simulink model "untitled"  (R2020a)
settings: Solver=VariableStepAuto  StartTime=0.0  StopTime=10.0  FixedStep=1e-10  RelTol=1e-3
libraries: powerlib x18, fuzblock x1, powerlib_meascontrol x1, re_lib x1
settings Model: Creator=Khojasteh Mirza  LastModifiedBy=Khojasteh Mirza

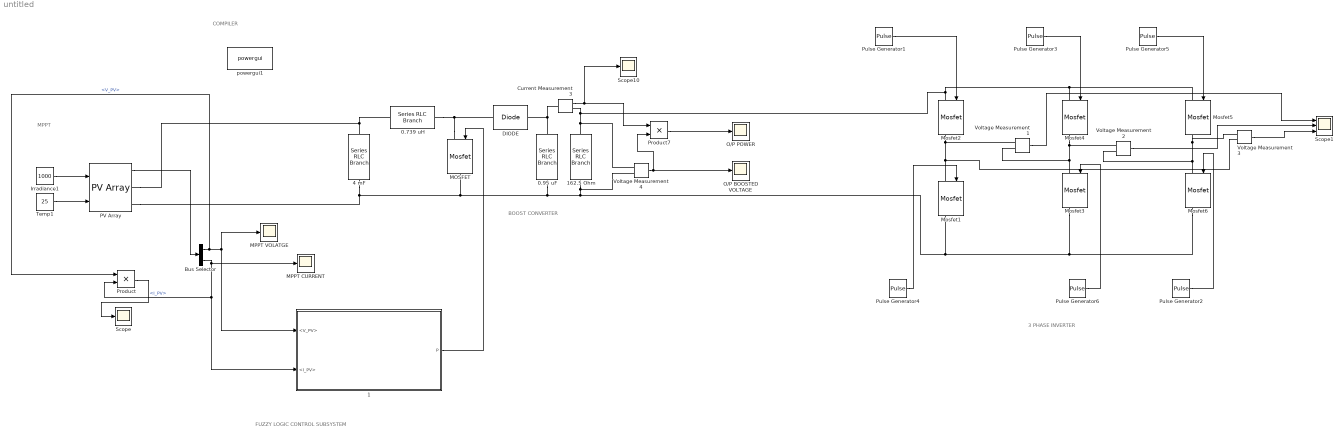
== system untitled ==
  note: 3 PHASE INVERTER
  note: BOOST CONVERTER
  note: FUZZY LOGIC CONTROL SUBSYSTEM
  note: COMPILER
  note: MPPT
  0.739 uH : powerlib/Elements/Series RLC Branch  LConnTagsString=__new0  RConnTagsString=__new0  BranchType=L  Resistance=1  Inductance=7.39e-5  SetiL0=off  InitialCurrent=0  Capacitance=1e-6  Setx0=off  InitialVoltage=0  Measurements=None
  0.95 uF : powerlib/Elements/Series RLC Branch  LConnTagsString=__new0  RConnTagsString=__new0  BranchType=C  Resistance=1  Inductance=1e-3  SetiL0=off  InitialCurrent=0  Capacitance=9.5e-5  Setx0=off  InitialVoltage=0  Measurements=None
  1 : Subsystem
  162.5 Ohm : powerlib/Elements/Series RLC Branch  LConnTagsString=__new0  RConnTagsString=__new0  BranchType=R  Resistance=162.5  Inductance=922.8515625e-6  SetiL0=off  InitialCurrent=0  Capacitance=1e-6  Setx0=off  InitialVoltage=0  Measurements=None
  4 mF : powerlib/Elements/Series RLC Branch  LConnTagsString=__new0  RConnTagsString=__new0  BranchType=C  Resistance=1  Inductance=1e-3  SetiL0=off  InitialCurrent=0  Capacitance=4000e-6  Setx0=off  InitialVoltage=0  Measurements=None
  Bus Selector : BusSelector  OutputSignals=V_PV,I_PV
  Current Measurement3 : powerlib/Measurements/Current Measurement  PhasorSimulation=off  OutputType=Complex  PSBequivalent=0
  DIODE : powerlib/Power Electronics/Diode  Ron=0.001  Lon=0  Vf=0.8  IC=0  UseSnubber=0  Rs=500  Cs=250e-9  Measurements=off
  Irradiance1 : Constant  Value=1000
  MOSFET : powerlib/Power Electronics/Mosfet  Ron=0.1  Lon=0  Rd=0.01  Vfd=0  IC=0  Rs=1e5  Cs=inf  Measurements=off
  MPPT CURRENT : Scope
  MPPT VOLATGE : Scope
  Mosfet{1..6} (6 alike) : powerlib/Power Electronics/Mosfet  Ron=0.1  Lon=0  Rd=0.01  Vfd=0  IC=0  Rs=1e5  Cs=inf  Measurements=on
  O/P BOOSTED VOLTAGE : Scope
  O/P POWER : Scope
  PV Array : re_lib/Solar/PV Array  Npar=1  Nser=1  PlotType=array @ 25 deg.C & specified irradiances  S_vec=[1000]  Temp_C_vec=[800]  ModuleName=Kyocera Solar KC200GT  PlotWhenSelected=off  Pm=200.143  Ncell=54  Voc=32.9  Isc=8.21  Vm=26.3  Im=7.61  beta_Voc_pc=-0.35502  alpha_Isc_pc=0.06  beta_Voc=-0.1168  alpha_Isc=0.004926  IL=8.2288  I0=2.3246e-10  nI=0.97736  Rsh=150.6921  Rs=0.34483  RobustModel=off  RobustCellTemperature=25  BAL=on  Tc=1e-6  Tfilter=5e-5
  Product : Product
  Product7 : Product
  Pulse Generator1 : DiscretePulseGenerator  PulseType=Time based  Period=0.02  PulseWidth=50
  Pulse Generator2 : DiscretePulseGenerator  PulseType=Time based  Period=0.02  PulseWidth=50  PhaseDelay=1/300
  Pulse Generator3 : DiscretePulseGenerator  PulseType=Time based  Period=0.02  PulseWidth=50  PhaseDelay=2/300
  Pulse Generator4 : DiscretePulseGenerator  PulseType=Time based  Period=0.02  PulseWidth=50  PhaseDelay=3/300
  Pulse Generator5 : DiscretePulseGenerator  PulseType=Time based  Period=0.02  PulseWidth=50  PhaseDelay=4/300
  Pulse Generator6 : DiscretePulseGenerator  PulseType=Time based  Period=0.02  PulseWidth=50  PhaseDelay=5/300
  Scope : Scope
  Scope1 : Scope  NumInputPorts=3
  Scope10 : Scope
  Temp1 : Constant  Value=25
  Voltage Measurement{1..4} (4 alike) : powerlib/Measurements/Voltage Measurement  PhasorSimulation=off  OutputType=Complex  PSBequivalent=0
  powergui1 : powerlib/powergui  Priority=1  SimulationMode=Continuous  SampleTime=5e-6  frequency=60  Iterations=50  frequencyindice=0  Pbase=100e6  ErrMax=1e-4  UnitsV=kV  UnitsW=MW  buscounter=0  FunctionMessages=off  echomessages=off  EnableUseOfTLC=off  CurrentSourceSwitches=off  DisableSnubberDevices=off  DisableRonSwitches=off  DisableVfSwitches=off  DisplayEquations=off  AutomaticDiscreteSolvers=off  SolverType=Tustin/Backward Euler (TBE)  Interpol=off  ExternalGateDelay=off  methode=off  Ts=100  x0status=blocks  SPID=on  SwTol=0  HookPort=off  NonlinearTolerance=1e-4  nMaxIteration=100  ContinueOnMaxIteration=off  RestoreLinks=warning  ResistiveCurrentMeasurement=off  Frange=[0:2:500]  Ylog=off  Xlog=on  ShowGrid=off  save=off  variable=ZData  structure=0  ZoomFFT=off  StartTime=0.0  cycles=1  DisplayStyle=1  fundamental=60  FreqAxis=off  MaxFrequency=1000  frequencyindicesteady=1  RmsSteady=1  display=off
  wires:
  Pulse Generator1/1 -> Mosfet2/1
  Pulse Generator2/1 -> Mosfet6/1
  Pulse Generator3/1 -> Mosfet4/1
  Pulse Generator4/1 -> Mosfet1/1
  Pulse Generator5/1 -> Mosfet5/1
  Pulse Generator6/1 -> Mosfet3/1
  Voltage Measurement1/1 -> Scope1/1
  Voltage Measurement2/1 -> Scope1/2
  Voltage Measurement3/1 -> Scope1/3
  Temp1/1 -> PV Array/2
  Product7/1 -> O/P POWER/1
  Irradiance1/1 -> PV Array/1
  Voltage Measurement4/1 -> Product7/2, O/P BOOSTED VOLTAGE/1
  Current Measurement3/1 -> Scope10/1, Product7/1
  PV Array/1 -> Bus Selector/1
  Bus Selector/1 -> Product/1, 1/1(<V_PV>), MPPT VOLATGE/1  "<V_PV>"
  Bus Selector/2 -> Product/2, 1/2(<I_PV>), MPPT CURRENT/1  "<I_PV>"
  1/1(P) -> MOSFET/1
  Product/1 -> Scope/1
  connections:
  Mosfet5/RConn1 -- Voltage Measurement2/LConn2 -- Mosfet6/LConn1 -- Voltage Measurement3/LConn1
  Mosfet4/RConn1 -- Voltage Measurement2/LConn1 -- Voltage Measurement1/LConn2 -- Mosfet3/LConn1
  Mosfet2/RConn1 -- Voltage Measurement3/LConn2 -- Mosfet1/LConn1 -- Voltage Measurement1/LConn1
  DIODE/RConn1 -- 0.95 uF/LConn1 -- Current Measurement3/LConn1
  PV Array/RConn1 -- 4 mF/LConn1 -- 0.739 uH/LConn1
  Mosfet6/RConn1 -- Mosfet3/RConn1 -- Voltage Measurement4/LConn2 -- 162.5 Ohm/RConn1 -- 4 mF/RConn1 -- PV Array/RConn2 -- MOSFET/RConn1 -- 0.95 uF/RConn1 -- Mosfet1/RConn1
  Mosfet5/LConn1 -- Mosfet4/LConn1 -- Current Measurement3/RConn1 -- Voltage Measurement4/LConn1 -- 162.5 Ohm/LConn1 -- Mosfet2/LConn1
  MOSFET/LConn1 -- 0.739 uH/RConn1 -- DIODE/LConn1

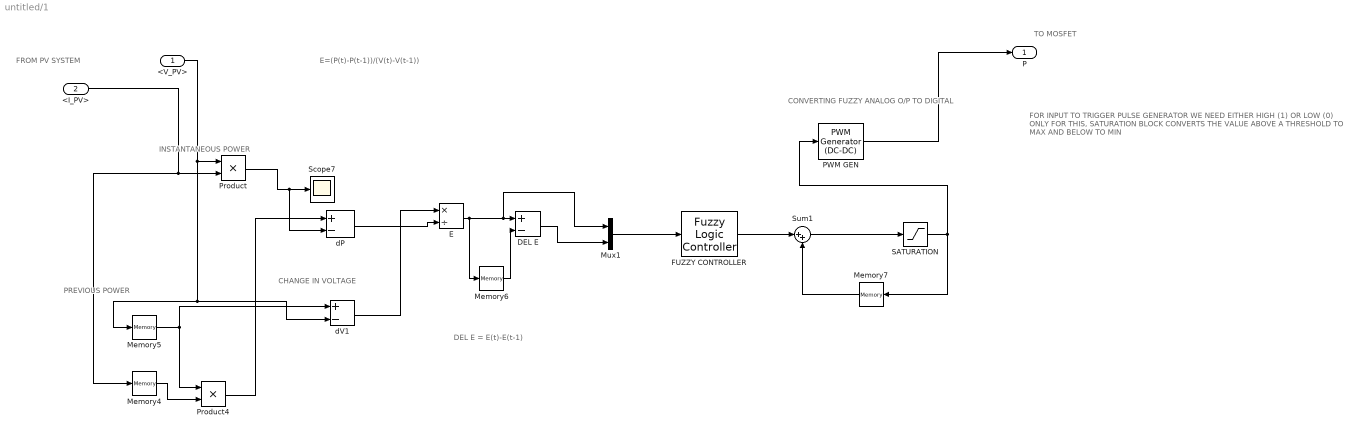
== system untitled/1 ==
  note: TO MOSFET
  note: FROM PV SYSTEM
  note: CONVERTING FUZZY ANALOG O/P TO DIGITAL
  note: CHANGE IN VOLTAGE
  note: PREVIOUS POWER
  note: INSTANTANEOUS POWER
  note: E=(P(t)-P(t-1))/(V(t)-V(t-1))
  note: DEL E = E(t)-E(t-1)
  note: FOR INPUT TO TRIGGER PULSE GENERATOR
      | WE NEED EITHER HIGH (1) OR LOW (0) ONLY
      |
      | FOR THIS, SATURATION BLOCK CONVERTS
      | THE VALUE ABOVE A THRESHOLD TO MAX AND BELOW
      | TO MIN
  <V_PV> : Inport
  <I_PV> : Inport  Port=2
  DEL E : Sum  Inputs=+-
  E : Product  Inputs=*/
  FUZZY CONTROLLER : fuzblock/Fuzzy Logic  Controller  FIS='fuzzy_mppt.fis'  OutputSampleNumber=101  DataType=double  FuzzifiedInputs=off  RuleFiringStrengths=off  RuleOutputs=off  AggregatedOutputs=off  SimulateUsing=Interpreted execution  OutOfRangeInputValueMessage=warning  NoRuleFiredMessage=warning  EmptyOutputFuzzySetMessage=warning
  Memory{4..7} (4 alike) : Memory
  Mux1 : Mux  Inputs=2
  PWM GEN : powerlib_meascontrol/Pulse & Signal Generators/PWM Generator (DC-DC)  Fsw=5000  Ts=0
  Product : Product
  Product4 : Product
  SATURATION : Saturate
  Scope7 : Scope
  Sum1 : Sum  Inputs=|++
  dP : Sum  Inputs=+-
  dV1 : Sum  Inputs=+-
  P : Outport
  wires:
  PWM GEN/1 -> P/1
  Memory5/1 -> dV1/1, Product4/1
  dV1/1 -> E/1
  E/1 -> Memory6/1, Mux1/1, DEL E/1
  FUZZY CONTROLLER/1 -> Sum1/1
  Memory7/1 -> Sum1/2
  Sum1/1 -> SATURATION/1
  DEL E/1 -> Mux1/2
  Product/1 -> dP/2, Scope7/1
  dP/1 -> E/2
  Memory6/1 -> DEL E/2
  <V_PV>/1 -> dV1/2, Memory5/1, Product/1
  Product4/1 -> dP/1
  Memory4/1 -> Product4/2
  <I_PV>/1 -> Product/2, Memory4/1
  SATURATION/1 -> PWM GEN/1, Memory7/1
  Mux1/1 -> FUZZY CONTROLLER/1
